simulink model "Transitions5_2018a"  (R2018a)
settings: Solver=VariableStepAuto  StartTime=0.0  StopTime=0.1  RelTol=1e-3
settings Model: Creator=BEAR  LastModifiedBy=bzhan

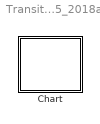
== system Transitions5_2018a ==
  Chart : Stateflow chart  TreatAsAtomicUnit=on

== stateflow chart Transitions5_2018a/Chart ==
  settings: updateMethod=DISCRETE  sampleTime=0.1
  state S
    en: f("enS")
    du: f("duS")
    state A
      en: f("enA")
      ex: f("exA")
    state B
      en: f("enB")
      ex: f("exB")
    S -> S : {f("condInner")}/{f("tranInner")}
    (default) -> A
    A -> B
    B -> A
  (default) -> S
  data: s function_input
  function f(s):
    | function f(s)
    |   fprintf(s+"\n");
